simulink library "MBDS_Subsystems"  (R2018b)
(part 13 of 15)

  in_DIAG_DigitalOutputsSTATIC.OUT_01_TD_DIAG/1 -> [u16Out_01_TD_DIAG], out_OUT_PCAN.Tx_Out.Out_01_Sts.Out_TD_DIAG/1
  in_IN_DigitalOutputsSTATIC.OUT_01_TD/1 -> [boOut_01_TD], out_OUT_PCAN.Tx_Out.Out_01_Sts.Out_TD/1
  in_IN_DigitalOutputsSTATIC.OUT_01_SENSE/1 -> out_OUT_PCAN.Tx_Out.Out_01_Sts.Out_SENSE/1
  in_DIAG_DigitalOutputsSTATIC.OUT_01_DIAG/1 -> out_OUT_PCAN.Tx_Out.Out_01_Sts.Out_DIAG/1, [boOut_01_DIAG]
  in_DIAG_DigitalOutputsSTATIC.OUT_12_TD_DIAG/1 -> [u16Out_12_TD_DIAG], out_OUT_PCAN.Tx_Out.Out_12_Sts.Out_TD_DIAG/1
  in_IN_DigitalOutputsSTATIC.OUT_12_TD/1 -> [boOut_12_TD], out_OUT_PCAN.Tx_Out.Out_12_Sts.Out_TD/1
  in_IN_DigitalOutputsSTATIC.OUT_12_SENSE/1 -> out_OUT_PCAN.Tx_Out.Out_12_Sts.Out_SENSE/1
  in_DIAG_DigitalOutputsSTATIC.OUT_12_DIAG/1 -> out_OUT_PCAN.Tx_Out.Out_12_Sts.Out_DIAG/1, [boOut_12_DIAG]
  in_IN_DigitalOutputsSTATIC.OUT_11_SENSE/1 -> out_OUT_PCAN.Tx_Out.Out_11_Sts.Out_SENSE/1
  in_DIAG_DigitalOutputsSTATIC.OUT_11_DIAG/1 -> out_OUT_PCAN.Tx_Out.Out_11_Sts.Out_DIAG/1, [boOut_11_DIAG]
  in_IN_DigitalOutputsSTATIC.OUT_10_SENSE/1 -> out_OUT_PCAN.Tx_Out.Out_10_Sts.Out_SENSE/1
  in_DIAG_DigitalOutputsSTATIC.OUT_10_DIAG/1 -> out_OUT_PCAN.Tx_Out.Out_10_Sts.Out_DIAG/1, [boOut_10_DIAG]
  [boSendEnable] -> out_OUT_PCAN.Tx_Out.Out_01_TD_Sts.MessageEnable/1, out_OUT_PCAN.Tx_Out.Out_02_Sts.MessageEnable/1, out_OUT_PCAN.Tx_Out.Out_03_Sts.MessageEnable/1, out_OUT_PCAN.Tx_Out.Out_04_Sts.MessageEnable/1, out_OUT_PCAN.Tx_Out.Out_04_TD_Sts.MessageEnable/1, out_OUT_PCAN.Tx_Out.Out_05_Sts.MessageEnable/1, out_OUT_PCAN.Tx_Out.Out_06_Sts.MessageEnable/1, out_OUT_PCAN.Tx_Out.Out_06_TD_Sts.MessageEnable/1, out_OUT_PCAN.Tx_Out.Out_07_Sts.MessageEnable/1, out_OUT_PCAN.Tx_Out.Out_07_TD_Sts.MessageEnable/1, out_OUT_PCAN.Tx_Out.Out_08_Sts.MessageEnable/1, out_OUT_PCAN.Tx_Out.Out_08_TD_Sts.MessageEnable/1, out_OUT_PCAN.Tx_Out.Out_09_Sts.MessageEnable/1, out_OUT_PCAN.Tx_Out.Out_10_Sts.MessageEnable/1, out_OUT_PCAN.Tx_Out.Out_11_Sts.MessageEnable/1, out_OUT_PCAN.Tx_Out.Out_12_Sts.MessageEnable/1, out_OUT_PCAN.Tx_Out.Out_12_TD_Sts.MessageEnable/1, out_OUT_PCAN.Tx_Out.Out_13_Sts.MessageEnable/1, out_OUT_PCAN.Tx_Out.Out_13_TD_Sts.MessageEnable/1, out_OUT_PCAN.Tx_Out.Out_14_Sts.MessageEnable/1, out_OUT_PCAN.Tx_Out.Out_14_TD_Sts.MessageEnable/1, out_OUT_PCAN.Tx_Out.Out_15_Sts.MessageEnable/1, out_OUT_PCAN.Tx_Out.Out_15_TD_Sts.MessageEnable/1, out_OUT_PCAN.Tx_Out.Out_16_Sts.MessageEnable/1, out_OUT_PCAN.Tx_Out.Out_17_Sts.MessageEnable/1, out_OUT_PCAN.Tx_Out.Out_19_Sts.MessageEnable/1, out_OUT_PCAN.Tx_Out.Out_01_Sts.MessageEnable/1
  bo_SendEnable/1 -> [boSendEnable]
  in_IN_DigitalOutputsSTATIC.OUT_09_SENSE/1 -> out_OUT_PCAN.Tx_Out.Out_09_Sts.Out_SENSE/1
  in_DIAG_DigitalOutputsSTATIC.OUT_09_DIAG/1 -> out_OUT_PCAN.Tx_Out.Out_09_Sts.Out_DIAG/1, [boOut_09_DIAG]
  in_DIAG_DigitalOutputsSTATIC.OUT_08_TD_DIAG/1 -> [u16Out_08_TD_DIAG], out_OUT_PCAN.Tx_Out.Out_08_Sts.Out_TD_DIAG/1
  in_IN_DigitalOutputsSTATIC.OUT_08_TD/1 -> [boOut_08_TD], out_OUT_PCAN.Tx_Out.Out_08_Sts.Out_TD/1
  in_IN_DigitalOutputsSTATIC.OUT_08_SENSE/1 -> out_OUT_PCAN.Tx_Out.Out_08_Sts.Out_SENSE/1
  in_DIAG_DigitalOutputsSTATIC.OUT_08_DIAG/1 -> out_OUT_PCAN.Tx_Out.Out_08_Sts.Out_DIAG/1, [boOut_08_DIAG]
  in_DIAG_DigitalOutputsSTATIC.OUT_07_TD_DIAG/1 -> [u16Out_07_TD_DIAG], out_OUT_PCAN.Tx_Out.Out_07_Sts.Out_TD_DIAG/1
  in_IN_DigitalOutputsSTATIC.OUT_07_TD/1 -> [boOut_07_TD], out_OUT_PCAN.Tx_Out.Out_07_Sts.Out_TD/1
  in_IN_DigitalOutputsSTATIC.OUT_07_SENSE/1 -> out_OUT_PCAN.Tx_Out.Out_07_Sts.Out_SENSE/1
  in_DIAG_DigitalOutputsSTATIC.OUT_07_DIAG/1 -> out_OUT_PCAN.Tx_Out.Out_07_Sts.Out_DIAG/1, [boOut_07_DIAG]
  in_IN_DigitalOutputsSTATIC.OUT_06_TD/1 -> [boOut_06_TD], out_OUT_PCAN.Tx_Out.Out_06_Sts.Out_TD/1
  in_DIAG_DigitalOutputsSTATIC.OUT_06_TD_DIAG/1 -> [u16Out_06_TD_DIAG], out_OUT_PCAN.Tx_Out.Out_06_Sts.Out_TD_DIAG/1
  in_IN_DigitalOutputsSTATIC.OUT_06_SENSE/1 -> out_OUT_PCAN.Tx_Out.Out_06_Sts.Out_SENSE/1
  in_DIAG_DigitalOutputsSTATIC.OUT_06_DIAG/1 -> out_OUT_PCAN.Tx_Out.Out_06_Sts.Out_DIAG/1, [boOut_06_DIAG]
  in_IN_DigitalOutputsSTATIC.OUT_05_SENSE/1 -> out_OUT_PCAN.Tx_Out.Out_05_Sts.Out_SENSE/1
  in_DIAG_DigitalOutputsSTATIC.OUT_05_DIAG/1 -> out_OUT_PCAN.Tx_Out.Out_05_Sts.Out_DIAG/1, [boOut_05_DIAG]
  in_IN_DigitalOutputsSTATIC.OUT_04_TD/1 -> [boOut_04_TD], out_OUT_PCAN.Tx_Out.Out_04_Sts.Out_TD/1
  in_DIAG_DigitalOutputsSTATIC.OUT_04_TD_DIAG/1 -> [u16Out_04_TD_DIAG], out_OUT_PCAN.Tx_Out.Out_04_Sts.Out_TD_DIAG/1
  in_IN_DigitalOutputsSTATIC.OUT_04_SENSE/1 -> out_OUT_PCAN.Tx_Out.Out_04_Sts.Out_SENSE/1
  in_DIAG_DigitalOutputsSTATIC.OUT_04_DIAG/1 -> out_OUT_PCAN.Tx_Out.Out_04_Sts.Out_DIAG/1, [boOut_04_DIAG]
  in_IN_DigitalOutputsSTATIC.OUT_03_SENSE/1 -> out_OUT_PCAN.Tx_Out.Out_03_Sts.Out_SENSE/1
  in_DIAG_DigitalOutputsSTATIC.OUT_03_DIAG/1 -> out_OUT_PCAN.Tx_Out.Out_03_Sts.Out_DIAG/1, [boOut_03_DIAG]
  in_IN_DigitalOutputsSTATIC.OUT_02_SENSE/1 -> out_OUT_PCAN.Tx_Out.Out_02_Sts.Out_SENSE/1
  in_DIAG_DigitalOutputsSTATIC.OUT_02_DIAG/1 -> out_OUT_PCAN.Tx_Out.Out_02_Sts.Out_DIAG/1, [boOut_02_DIAG]
